simulink model "Example_Hydraulic_ValveFn"  (R2013b)
settings: Solver=ode45  StartTime=0.0  StopTime=210  RelTol=1e-3
libraries: carnot x4, simulink x1
settings Model: Creator=drhf  LastModifiedBy=drhf
settings OptimizationCC: ExpressionDepthLimit=2147483647
settings DebuggingCC: StateNameClashWarn=warning
settings GRTTargetCC: CombineOutputUpdateFcns=off  GRTInterface=on

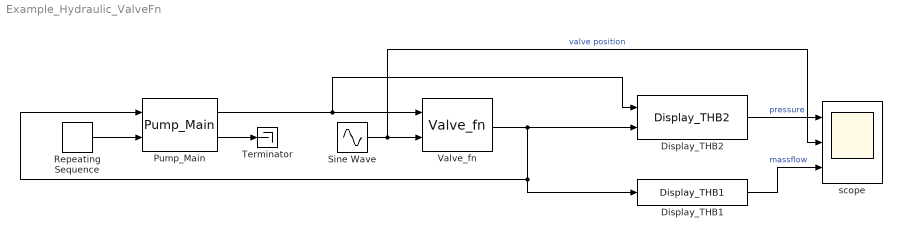
== system Example_Hydraulic_ValveFn ==
  Display_THB1 : carnot/Outputs/Display_THB1  t=off  m=on  p=off  id=off  mix=off  d=off
  Display_THB2 : carnot/Outputs/Display_THB2  t=off  m=off  p=on  id=off  mix=off  d=off
  Pump_Main : carnot/Hydraulics/Pump_Main  a0=2.7e4  a1=-1.2e4  a2=0%-3e-3  dia=0.025  t1=5  p0=3e5  IDchk=off  fluid_id=Water  mix=0  ua=1  mcp=500  tamb=20
  Repeating Sequence : simulink/Sources/Repeating Sequence  rep_seq_t=[0 20 60 200]  rep_seq_y=[0 0 1 1]
  Sine Wave : Sin  Amplitude=0.6  Bias=0.5  Frequency=1/20  SampleTime=0
  Terminator : Terminator
  Valve_fn : carnot/Hydraulics/Valve_fn  kv=0.7  kvs=0.9  op=0.5
  scope : Scope  NumInputPorts=3
      settings: TickLabels=on  YMin=0~-5~-5  YMax=5~5~5
  wires:
  Repeating Sequence/1 -> Pump_Main/2
  Pump_Main/2 -> Terminator/1
  Sine Wave/1 -> Valve_fn/2, scope/2  "valve position"
  Pump_Main/1 -> Valve_fn/1, Display_THB2/1
  Display_THB2/1 -> scope/1  "pressure"
  Valve_fn/1 -> Pump_Main/1, Display_THB1/1, Display_THB2/2
  Display_THB1/1 -> scope/3  "massflow"
